simulink model "NewModel"  (R2018a)
settings: Solver=VariableStepAuto  StartTime=0.0  StopTime=1  RelTol=1e-3
undefined symbols (not defined in the file): a22, a23, a24, a42, a43, a44, a66, b21, b22, b41, b42, b61, b62, F1, k1, k3, Lt1, Lt3
libraries: simulink x1
settings Model: Creator=Andrei  LastModifiedBy=Andrei

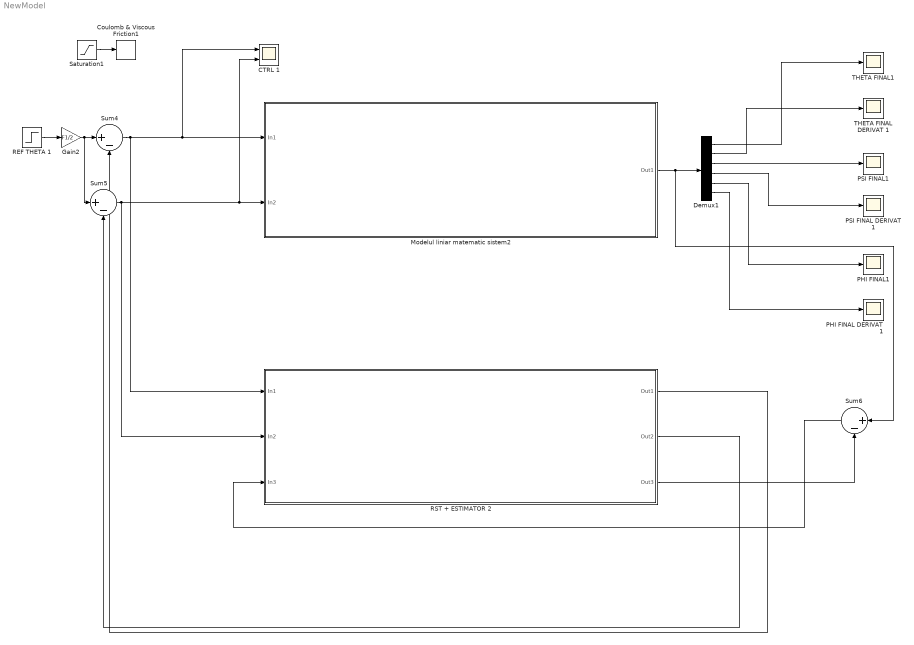
== system NewModel ==
  CTRL 1 : Scope  NumInputPorts=2
  Coulomb & Viscous Friction1 : simulink/Discontinuities/Coulomb & Viscous Friction  offset=0.055  gain=1
      settings: SourceProductName=Simulink
  Demux1 : Demux  Outputs=6
  Gain2 : Gain  Gain=F1/2
  Modelul liniar matematic sistem2 : Subsystem
  PHI FINAL DERIVAT 1 : Scope
  PHI FINAL1 : Scope
  PSI FINAL DERIVAT 1 : Scope
  PSI FINAL1 : Scope
  REF THETA 1 : Step  Time=0  SampleTime=0
  RST + ESTIMATOR 2 : Subsystem
  Saturation1 : Saturate  UpperLimit=0.6  LowerLimit=-0.6
  Sum4 : Sum  Inputs=|+-
  Sum5 : Sum  Inputs=|+-
  Sum6 : Sum  Inputs=|+-
  THETA FINAL DERIVAT 1 : Scope
  THETA FINAL1 : Scope
  wires:
  Sum6/1 -> RST + ESTIMATOR 2/3(In3)
  Demux1/3 -> PSI FINAL1/1
  REF THETA 1/1 -> Gain2/1
  Sum5/1 -> CTRL 1/2, Modelul liniar matematic sistem2/2(In2), RST + ESTIMATOR 2/2(In2)
  RST + ESTIMATOR 2/2(Out2) -> Sum5/2
  RST + ESTIMATOR 2/3(Out3) -> Sum6/2
  Demux1/6 -> PHI FINAL DERIVAT 1/1
  Gain2/1 -> Sum5/1, Sum4/1
  Modelul liniar matematic sistem2/1(Out1) -> Sum6/1, Demux1/1
  Demux1/1 -> THETA FINAL1/1
  Demux1/2 -> THETA FINAL DERIVAT 1/1
  RST + ESTIMATOR 2/1(Out1) -> Sum4/2
  Demux1/4 -> PSI FINAL DERIVAT 1/1
  Saturation1/1 -> Coulomb & Viscous Friction1/1
  Demux1/5 -> PHI FINAL1/1
  Sum4/1 -> CTRL 1/1, Modelul liniar matematic sistem2/1(In1), RST + ESTIMATOR 2/1(In1)

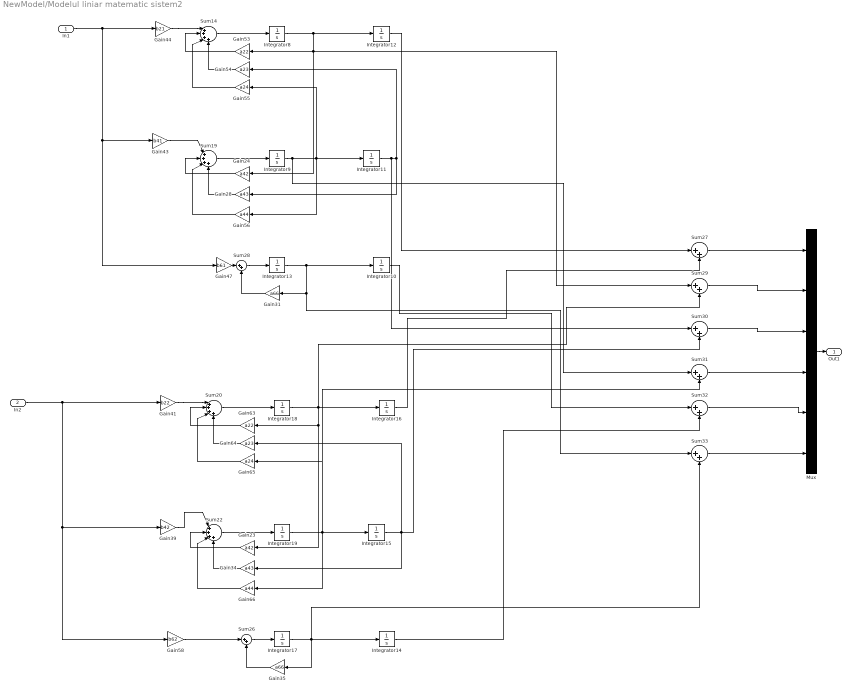
== system NewModel/Modelul liniar matematic sistem2 ==
  In1 : Inport
  In2 : Inport  Port=2
  Gain23 : Gain  Gain=a42
  Gain24 : Gain  Gain=a42
  Gain28 : Gain  Gain=a43
  Gain31 : Gain  Gain=a66
  Gain34 : Gain  Gain=a43
  Gain35 : Gain  Gain=a66
  Gain39 : Gain  Gain=b42
  Gain41 : Gain  Gain=b22
  Gain43 : Gain  Gain=b41
  Gain44 : Gain  Gain=b21
  Gain47 : Gain  Gain=b61
  Gain53 : Gain  Gain=a22
  Gain54 : Gain  Gain=a23
  Gain55 : Gain  Gain=a24
  Gain56 : Gain  Gain=a44
  Gain58 : Gain  Gain=b62
  Gain63 : Gain  Gain=a22
  Gain64 : Gain  Gain=a23
  Gain65 : Gain  Gain=a24
  Gain66 : Gain  Gain=a44
  Integrator{8..19} (12 alike) : Integrator
  Mux : Mux  Inputs=6
  Sum{14,19..20,22} (4 alike) : Sum  Inputs=|++++
  Sum{26..33} (8 alike) : Sum  Inputs=|++
  Out1 : Outport
  wires:
  Integrator9/1 -> Sum31/1, Gain56/1, Gain55/1, Integrator11/1
  Gain31/1 -> Sum28/2
  Gain66/1 -> Sum22/3
  Integrator19/1 -> Integrator15/1, Sum31/2, Gain66/1, Gain65/1
  Sum32/1 -> Mux/5
  Gain39/1 -> Sum22/1
  Gain55/1 -> Sum14/3
  Sum20/1 -> Integrator18/1
  Sum14/1 -> Integrator8/1
  Integrator17/1 -> Gain35/1, Integrator14/1, Sum33/2
  Sum30/1 -> Mux/3
  Gain44/1 -> Sum14/1
  Integrator8/1 -> Gain24/1, Sum29/1, Gain53/1, Integrator12/1
  Sum22/1 -> Integrator19/1
  Mux/1 -> Out1/1
  Integrator18/1 -> Sum29/2, Gain23/1, Gain63/1, Integrator16/1
  Gain24/1 -> Sum19/2
  Gain53/1 -> Sum14/2
  Sum19/1 -> Integrator9/1
  Sum33/1 -> Mux/6
  Gain64/1 -> Sum20/4
  Integrator14/1 -> Sum32/2
  Gain54/1 -> Sum14/4
  Integrator11/1 -> Sum30/1, Gain54/1, Gain28/1
  Integrator13/1 -> Sum33/1, Gain31/1, Integrator10/1
  Gain41/1 -> Sum20/1
  Gain34/1 -> Sum22/4
  Sum27/1 -> Mux/1
  Integrator16/1 -> Sum27/2
  Integrator15/1 -> Sum30/2, Gain64/1, Gain34/1
  Gain28/1 -> Sum19/4
  Gain47/1 -> Sum28/1
  Sum28/1 -> Integrator13/1
  Gain43/1 -> Sum19/1
  Gain35/1 -> Sum26/2
  Gain63/1 -> Sum20/2
  Gain23/1 -> Sum22/2
  Sum31/1 -> Mux/4
  Sum29/1 -> Mux/2
  Integrator12/1 -> Sum27/1
  Gain65/1 -> Sum20/3
  Gain56/1 -> Sum19/3
  Integrator10/1 -> Sum32/1
  Sum26/1 -> Integrator17/1
  Gain58/1 -> Sum26/1
  In1/1 -> Gain47/1, Gain43/1, Gain44/1
  In2/1 -> Gain39/1, Gain58/1, Gain41/1

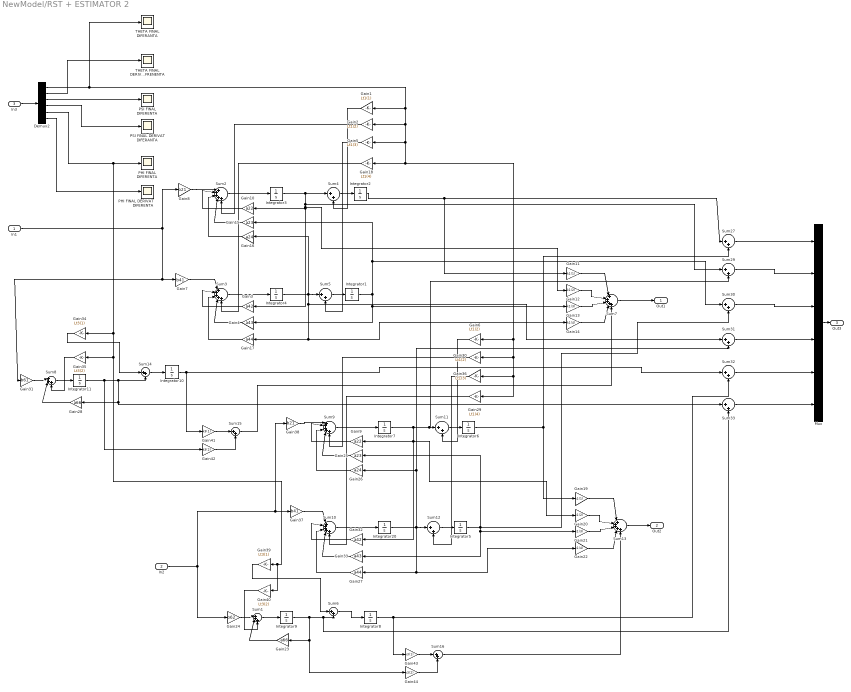
== system NewModel/RST + ESTIMATOR 2 ==
  In1 : Inport
  In2 : Inport  Port=2
  In3 : Inport  Port=3
  Demux2 : Demux  Outputs=6
  Gain1 : Gain  Gain=Lt1(1)
  Gain10 : Gain  Gain=a22
  Gain11 : Gain  Gain=k1(1)
  Gain12 : Gain  Gain=k1(2)
  Gain13 : Gain  Gain=k1(3)
  Gain14 : Gain  Gain=k1(4)
  Gain15 : Gain  Gain=a23
  Gain16 : Gain  Gain=a24
  Gain17 : Gain  Gain=a44
  Gain18 : Gain  Gain=Lt1(4)
  Gain19 : Gain  Gain=k1(1)
  Gain2 : Gain  Gain=Lt1(2)
  Gain20 : Gain  Gain=k1(2)
  Gain21 : Gain  Gain=k1(3)
  Gain22 : Gain  Gain=k1(4)
  Gain23 : Gain  Gain=a66
  Gain24 : Gain  Gain=b62
  Gain25 : Gain  Gain=a23
  Gain26 : Gain  Gain=a24
  Gain27 : Gain  Gain=a44
  Gain28 : Gain  Gain=a66
  Gain29 : Gain  Gain=Lt1(4)
  Gain3 : Gain  Gain=a42
  Gain30 : Gain  Gain=Lt1(2)
  Gain31 : Gain  Gain=b61
  Gain32 : Gain  Gain=a42
  Gain33 : Gain  Gain=a43
  Gain34 : Gain  Gain=Lt3(1)
  Gain35 : Gain  Gain=Lt3(2)
  Gain36 : Gain  Gain=Lt1(3)
  Gain37 : Gain  Gain=b41
  Gain38 : Gain  Gain=b21
  Gain39 : Gain  Gain=Lt3(1)
  Gain4 : Gain  Gain=a43
  Gain40 : Gain  Gain=Lt3(2)
  Gain41 : Gain  Gain=k3(1)
  Gain42 : Gain  Gain=k3(2)
  Gain43 : Gain  Gain=k3(1)
  Gain44 : Gain  Gain=k3(2)
  Gain5 : Gain  Gain=Lt1(3)
  Gain6 : Gain  Gain=Lt1(2)
  Gain7 : Gain  Gain=b41
  Gain8 : Gain  Gain=b21
  Gain9 : Gain  Gain=a22
  Integrator{1..11,20} (12 alike) : Integrator
  Mux : Mux  Inputs=6
  PHI FINAL DERIVAT DIFERENTA : Scope
  PHI FINAL DIFERENTA : Scope
  PSI FINAL DERIVAT DIFERANTA : Scope
  PSI FINAL DIFERENTA : Scope
  Sum1 : Sum  Inputs=|+++
  Sum{2..3,7,9..10,13} (6 alike) : Sum  Inputs=|+++++
  Sum{4..6,11..12,14..16,27,29..33} (14 alike) : Sum  Inputs=|++
  Sum8 : Sum  Inputs=|+++
  THETA FINAL DERIVAT DIFRENENTA : Scope
  THETA FINAL DIFERANTA : Scope
  Out1 : Outport
  Out2 : Outport  Port=2
  Out3 : Outport  Port=3
  wires:
  Integrator5/1 -> Gain33/1, Gain21/1, Gain25/1, Sum30/2
  Sum9/1 -> Integrator7/1
  Sum13/1 -> Out2/1
  Gain9/1 -> Sum9/2
  Gain38/1 -> Sum9/1
  Sum10/1 -> Integrator20/1
  Sum12/1 -> Integrator5/1
  Integrator7/1 -> Sum11/1, Sum29/2, Gain20/1, Gain32/1, Gain9/1
  Gain25/1 -> Sum9/4
  Gain37/1 -> Sum10/1
  Sum7/1 -> Out1/1
  Demux2/1 -> Gain29/1, Gain36/1, Gain30/1, Gain6/1, Gain18/1, Gain5/1, Gain2/1, Gain1/1, THETA FINAL DIFERANTA/1
  Integrator6/1 -> Gain19/1, Sum27/2
  Gain22/1 -> Sum13/4
  Gain30/1 -> Sum9/5
  Gain32/1 -> Sum10/2
  Gain36/1 -> Sum12/2
  Integrator20/1 -> Gain26/1, Sum31/2, Gain22/1, Gain27/1, Sum12/1
  Gain19/1 -> Sum13/1
  Gain20/1 -> Sum13/2
  Gain33/1 -> Sum10/4
  Sum11/1 -> Integrator6/1
  Gain21/1 -> Sum13/3
  Gain29/1 -> Sum10/5
  Gain8/1 -> Sum2/1
  Sum3/1 -> Integrator4/1
  Integrator3/1 -> Gain12/1, Gain3/1, Gain10/1, Sum29/1, Sum4/1
  Sum5/1 -> Integrator1/1
  Gain5/1 -> Sum5/2
  Gain3/1 -> Sum3/2
  Gain2/1 -> Sum2/5
  Gain14/1 -> Sum7/4
  Integrator2/1 -> Gain11/1, Sum27/1
  Gain13/1 -> Sum7/3
  Gain4/1 -> Sum3/4
  Sum4/1 -> Integrator2/1
  Gain26/1 -> Sum9/3
  Gain12/1 -> Sum7/2
  Integrator4/1 -> Sum31/1, Gain14/1, Gain17/1, Sum5/1, Gain16/1
  Gain11/1 -> Sum7/1
  Gain18/1 -> Sum3/5
  Gain16/1 -> Sum2/3
  Gain17/1 -> Sum3/3
  Gain1/1 -> Sum4/2
  Sum2/1 -> Integrator3/1
  Gain15/1 -> Sum2/4
  Integrator1/1 -> Gain15/1, Sum30/1, Gain4/1, Gain13/1
  Gain27/1 -> Sum10/3
  Gain7/1 -> Sum3/1
  Gain10/1 -> Sum2/2
  Gain6/1 -> Sum11/2
  In2/1 -> Gain38/1, Gain37/1, Gain24/1
  Sum30/1 -> Mux/3
  Sum31/1 -> Mux/4
  Sum27/1 -> Mux/1
  Sum32/1 -> Mux/5
  Sum29/1 -> Mux/2
  Sum33/1 -> Mux/6
  Mux/1 -> Out3/1
  In1/1 -> Gain31/1, Gain7/1, Gain8/1
  Sum1/1 -> Integrator9/1
  Gain24/1 -> Sum1/1
  Gain23/1 -> Sum1/2
  Integrator9/1 -> Sum6/2, Sum33/2, Gain44/1, Gain23/1
  Sum6/1 -> Integrator8/1
  Integrator11/1 -> Gain42/1, Sum14/2, Sum33/1, Gain28/1
  Sum8/1 -> Integrator11/1
  Gain28/1 -> Sum8/2
  Sum14/1 -> Integrator10/1
  Gain31/1 -> Sum8/1
  Gain39/1 -> Sum6/1
  Gain40/1 -> Sum1/3
  Gain34/1 -> Sum14/1
  Gain35/1 -> Sum8/3
  Integrator10/1 -> Gain41/1, Sum32/1
  Integrator8/1 -> Gain43/1, Sum32/2
  Gain41/1 -> Sum15/1
  Gain42/1 -> Sum15/2
  Gain44/1 -> Sum16/2
  Gain43/1 -> Sum16/1
  Demux2/2 -> THETA FINAL DERIVAT DIFRENENTA/1
  Demux2/5 -> Gain40/1, Gain39/1, Gain35/1, Gain34/1, PHI FINAL DIFERENTA/1
  Demux2/3 -> PSI FINAL DIFERENTA/1
  Demux2/6 -> PHI FINAL DERIVAT DIFERENTA/1
  Demux2/4 -> PSI FINAL DERIVAT DIFERANTA/1
  In3/1 -> Demux2/1
  Sum15/1 -> Sum7/5
  Sum16/1 -> Sum13/5
